simulink model "quatSim"  (R2016a)
settings: Solver=FixedStepAuto  StartTime=0.0  StopTime=79.38  FixedStep=1/100  RelTol=1e-3
model workspace: external: MAT-File config.mat (data not in the file)
values from neighbouring files (symbols this model uses):
  initialCondition = [1 0 0 0 0.00972301529379 -0.0766046660947 -0.0114540485936]    [config.mat]    (also in estimatorTest.m = [     1; kalmanEstimator.m = [1;0;0;0;y_valid(1,1:3)'])
settings Model: Creator=combine  LastModifiedBy=combine

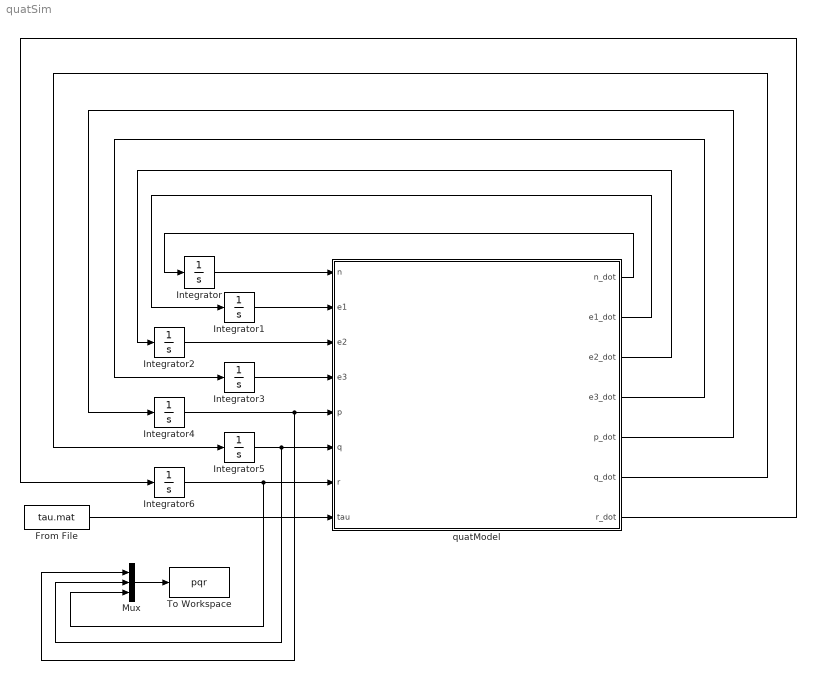
== system quatSim ==
  From File : FromFile  FileName=tau.mat  SampleTime=0
  Integrator : Integrator  InitialCondition=initialCondition(1)  ContinuousStateAttributes='n'
  Integrator1 : Integrator  InitialCondition=initialCondition(2)  ContinuousStateAttributes='e1'
  Integrator2 : Integrator  InitialCondition=initialCondition(3)  ContinuousStateAttributes='e2'
  Integrator3 : Integrator  InitialCondition=initialCondition(4)  ContinuousStateAttributes='e3'
  Integrator4 : Integrator  InitialCondition=initialCondition(5)  ContinuousStateAttributes='p'
  Integrator5 : Integrator  InitialCondition=initialCondition(6)  ContinuousStateAttributes='q'
  Integrator6 : Integrator  InitialCondition=initialCondition(7)  ContinuousStateAttributes='r'
  Mux : Mux  Inputs=3
  To Workspace : ToWorkspace  VariableName=pqr  SaveFormat=Timeseries  SampleTime=-1
  quatModel : MATLAB Function  TreatAsAtomicUnit=on
  wires:
  Integrator/1 -> quatModel/1(n)
  Integrator1/1 -> quatModel/2(e1)
  Integrator2/1 -> quatModel/3(e2)
  Integrator3/1 -> quatModel/4(e3)
  Integrator4/1 -> Mux/1, quatModel/5(p)
  Integrator5/1 -> Mux/2, quatModel/6(q)
  Integrator6/1 -> Mux/3, quatModel/7(r)
  quatModel/1(n_dot) -> Integrator/1
  quatModel/2(e1_dot) -> Integrator1/1
  quatModel/3(e2_dot) -> Integrator2/1
  quatModel/4(e3_dot) -> Integrator3/1
  quatModel/5(p_dot) -> Integrator4/1
  quatModel/6(q_dot) -> Integrator5/1
  quatModel/7(r_dot) -> Integrator6/1
  From File/1 -> quatModel/8(tau)
  Mux/1 -> To Workspace/1

== matlab function quatSim/quatModel ==
  data: n input; n_dot output; e1 input; e2 input; e3 input; p input; q input; r input; tau input size=6; e1_dot output; e2_dot output; e3_dot output; p_dot output; q_dot output; r_dot output; EstimatedParams parameter
function [n_dot,e1_dot,e2_dot,e3_dot,p_dot,q_dot,r_dot] = quatModel(n,e1,e2,e3,p,q,r,tau,EstimatedParams)
%#codegen
m=6.621;%ROVmass[kg];
g=9.81744;%Gravity[m/s^2]
rho=1000;%waterdensity[kg/m^3]
V=0.012;%Discplacedwatervolume[m^3]
%ThrusterplacementfromCO[m]
lx1=0.16;
ly1=0.11;
ly2=0.11;
lx2=0.16;
ly3=0.11;
lx5=0.2;
ly4=0.11;
lz6=0.11;
B=m*g;
%extractforcesfromthrusters
f1=tau(1);
f2=tau(2);
f3=tau(3);
f4=tau(4);
f5=tau(5);
f6=tau(6);

zb          = EstimatedParams(1);
Kp          = EstimatedParams(2);
Kp_dot      = EstimatedParams(3);
Kp_abs_p    = EstimatedParams(4); 
Mq          = EstimatedParams(5);
Mq_dot      = EstimatedParams(6);
Mq_abs_q    = EstimatedParams(7);
Nr          = EstimatedParams(8);
Nr_dot      = EstimatedParams(9);
Nr_abs_r    = EstimatedParams(10);
Ix          = EstimatedParams(11);
Iy          = EstimatedParams(12);
Iz          = EstimatedParams(13);
Ix_Kp_dot   = EstimatedParams(14);
Iy_Mq_dot   = EstimatedParams(15);
Iz_Nr_dot   = EstimatedParams(16);


n_dot=- (e1*p)/2 - (e2*q)/2 - (e3*r)/2 - n*(50*e1^2 + 50*e2^2 + 50*e3^2 + 50*n^2 - 50);
e1_dot=   (e2*r)/2 - (e3*q)/2 + (n*p)/2 - e1*(50*e1^2 + 50*e2^2 + 50*e3^2 + 50*n^2 - 50);
e2_dot=   (e3*p)/2 - (e1*r)/2 + (n*q)/2 - e2*(50*e1^2 + 50*e2^2 + 50*e3^2 + 50*n^2 - 50);
e3_dot=   (e1*q)/2 - (e2*p)/2 + (n*r)/2 - e3*(50*e1^2 + 50*e2^2 + 50*e3^2 + 50*n^2 - 50);
p_dot=(f1*ly1-f2*ly2+f6*lz6+p*(Kp+Kp_abs_p*abs(p))-Mq_dot*q*r+Nr_dot*q*r+q*r*(Iy-Iz)+B*zb*(2*e2*e3+2*e1*n))/Ix_Kp_dot;
q_dot=(f1*lx1+f2*lx2-f5*lx5+q*(Mq+Mq_abs_q*abs(q))+Kp_dot*p*r-Nr_dot*p*r-p*r*(Ix-Iz)-B*zb*(2*e1*e3-2*e2*n))/Iy_Mq_dot;
r_dot=(r*(Nr+Nr_abs_r*abs(r))+f3*ly3-f4*ly4-Kp_dot*p*q+Mq_dot*p*q+p*q*(Ix-Iy))/Iz_Nr_dot;
